simulink model "hw1_sub"  (R2019a)
settings: Solver=VariableStepAuto  StartTime=0.0  StopTime=70  RelTol=1e-12
model workspace (MAT data in the model file):
  d_tar = 20
values from neighbouring files (symbols this model uses):
  d_0 = 8    [acc1.m]
  t_H_tar = 1    [acc1.m]
  v_H0 = 28    [acc1.m]
  v_L0 = 36    [acc1.m]
  v_tar = 36    [acc1.m]
  x_H0 = 0    [acc1.m]
  x_L0 = 50    [acc1.m]
undefined symbols (not defined in the file or in its folder): sigbuilder_block
libraries: cstblocks x3
settings Model: Creator=jake  LastModifiedBy=Lorenzo
settings DebuggingCC: SFMachineParentedDataDiag=error

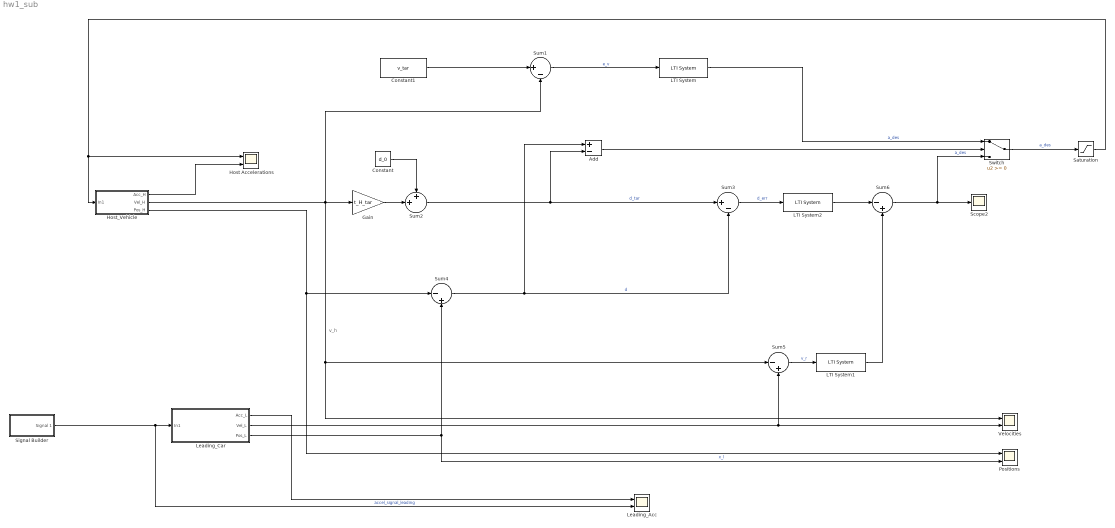
== system hw1_sub ==
  note: v_h
  Add : Sum  Inputs=+-
  Constant : Constant  Value=d_0
  Constant1 : Constant  Value=v_tar
  Gain : Gain  Gain=t_H_tar
  Host Accelerations : Scope  NumInputPorts=2
  Host_Vehicle : Subsystem
  LTI System : cstblocks/LTI System  sys=K_v  IC=[]
  LTI System1 : cstblocks/LTI System  sys=K_v_r  IC=[]
  LTI System2 : cstblocks/LTI System  sys=K_d_err  IC=[]
  Leading_Acc : Scope  NumInputPorts=2
  Leading_Car : Subsystem
  Positions : Scope  NumInputPorts=2
  Saturation : Saturate  UpperLimit=5  LowerLimit=-3
  Scope2 : Scope
  Signal Builder : Subsystem  Tag=STV Subsys  LoadFcn=sigbuilder_block('load');  StartFcn=sigbuilder_block('start');  StopFcn=sigbuilder_block('stop');  ClipboardFcn=sigbuilder_block('clipboard');  mask(Sigbuilder block){tuvar=[0:10]}
      mask help: Simulink:masks:SigbuilderBlock_MD
      mask init:
      | if ~strcmp(get_param(bdroot(gcbh),'SimulationStatus'),'stopped') tuvar = sigbuilder_block('maskInit'); end
      settings: CopyFcn=sigbuilder_block('copy');  DeleteFcn=sigbuilder_block('delete');  ModelCloseFcn=sigbuilder_block('modelClose');  PreSaveFcn=sigbuilder_block('preSave');  PauseFcn=sigbuilder_block('pause');  ContinueFcn=sigbuilder_block('continue');  NameChangeFcn=sigbuilder_block('namechange');  OpenFcn=sigbuilder_block('open',[303 126.6 843.6 459.6 ]);  CloseFcn=sigbuilder_block('close');
      mask Display: plot(0, 0, 100, 100,[2, 2, 32, 32, 2], [68, 8, 8, 68, 68],[32, 2], [38, 38], [32, 19, 2],[53, 60, 44], [32, 17, 17, 2],[16, 16, 31, 31]);txt = getActiveGroup(gcbh);text(2, 100, txt,'verticalAlignment', 'top');
  Sum1 : Sum  Inputs=|+-
  Sum2 : Sum  Inputs=++|
  Sum3 : Sum  Inputs=|+-
  Sum4 : Sum  Inputs=|-+
  Sum5 : Sum  Inputs=|-+
  Sum6 : Sum  Inputs=|-+
  Switch : Switch
  Velocities : Scope  NumInputPorts=2
  wires:
  Leading_Car/3(Pos_L) -> Positions/2, Sum4/2  "x_l"
  Sum1/1 -> LTI System/1  "e_v"
  Gain/1 -> Sum2/2
  Constant/1 -> Sum2/1
  Sum2/1 -> Add/2, Sum3/1  "d_tar"
  Sum4/1 -> Add/1, Sum3/2  "d"
  Sum5/1 -> LTI System1/1  "v_r"
  Sum3/1 -> LTI System2/1  "d_err"
  LTI System1/1 -> Sum6/2
  LTI System2/1 -> Sum6/1
  Sum6/1 -> Switch/3, Scope2/1  "a_des"
  LTI System/1 -> Switch/1  "a_des"
  Constant1/1 -> Sum1/1
  Switch/1 -> Saturation/1  "a_des"
  Signal Builder/1(Signal 1) -> Leading_Acc/2, Leading_Car/1(In1)  "accel_signal_leading"
  Add/1 -> Switch/2
  Leading_Car/2(Vel_L) -> Sum5/2, Velocities/2
  Leading_Car/1(Acc_L) -> Leading_Acc/1
  Host_Vehicle/2(Vel_H) -> Sum5/1, Velocities/1, Sum1/2, Gain/1
  Host_Vehicle/3(Pos_H) -> Positions/1, Sum4/1
  Saturation/1 -> Host Accelerations/1, Host_Vehicle/1(In1)
  Host_Vehicle/1(Acc_H) -> Host Accelerations/2

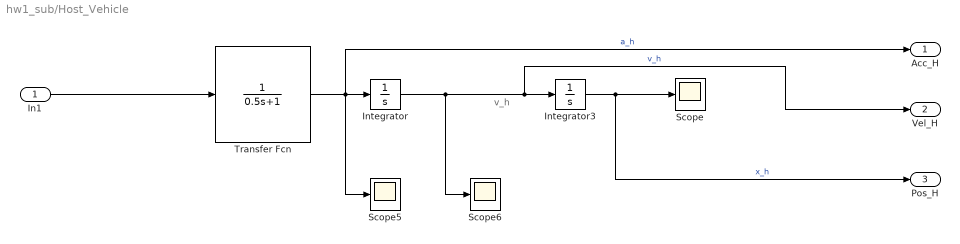
== system hw1_sub/Host_Vehicle ==
  note: v_h
  In1 : Inport
  Integrator : Integrator  InitialCondition=v_H0
  Integrator3 : Integrator  InitialCondition=x_H0
  Scope : Scope
  Scope5 : Scope
  Scope6 : Scope
  Transfer Fcn : TransferFcn  Denominator=[0.5 1]
  Acc_H : Outport
  Vel_H : Outport  Port=2
  Pos_H : Outport  Port=3
  wires:
  Integrator3/1 -> Pos_H/1, Scope/1  "x_h"
  Integrator/1 -> Scope6/1, Vel_H/1, Integrator3/1  "v_h"
  Transfer Fcn/1 -> Acc_H/1, Scope5/1, Integrator/1  "a_h"
  In1/1 -> Transfer Fcn/1

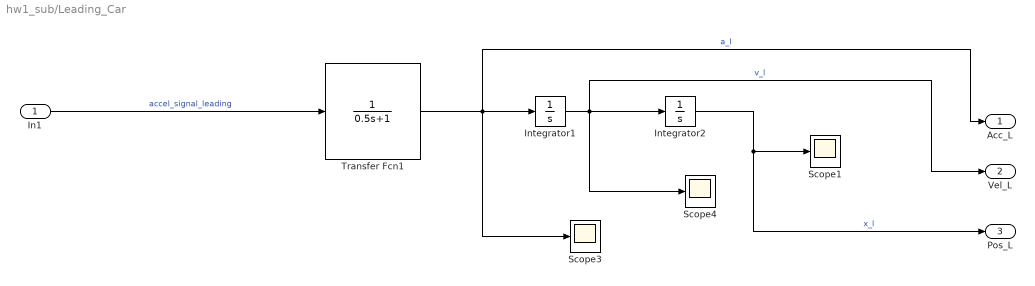
== system hw1_sub/Leading_Car ==
  In1 : Inport
  Integrator1 : Integrator  InitialCondition=v_L0
  Integrator2 : Integrator  InitialCondition=x_L0
  Scope1 : Scope
  Scope3 : Scope
  Scope4 : Scope
  Transfer Fcn1 : TransferFcn  Denominator=[0.5 1]
  Acc_L : Outport
  Vel_L : Outport  Port=2
  Pos_L : Outport  Port=3
  wires:
  Integrator1/1 -> Scope4/1, Vel_L/1, Integrator2/1  "v_l"
  Integrator2/1 -> Pos_L/1, Scope1/1  "x_l"
  Transfer Fcn1/1 -> Scope3/1, Acc_L/1, Integrator1/1  "a_l"
  In1/1 -> Transfer Fcn1/1  "accel_signal_leading"

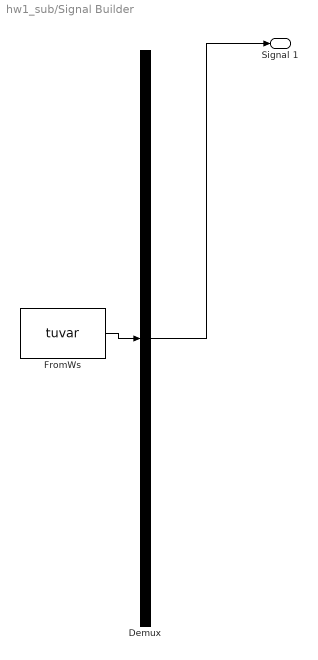
== system hw1_sub/Signal Builder ==
  Demux : Demux  Tag=STV Demux  Outputs=1
      settings: DisplayOption=none
  FromWs : FromWorkspace  Tag=STV FromWs  VariableName=tuvar
      SigBuilderData=|
      | common.afterFinalStr = 'Extrapolate'
      | common.sampleTime = 0
      | dataSet.timeRange = [0 46]
      | dataSet.name = 'Group 1'
      | sbobj.Groups.Name = 'Group 1'
      | sbobj.Groups.Signals.Name = 'Signal 1'
      | sbobj.Groups.Signals.XData = [0 10 10.5 13.5 14 40 40.5 43.5 44 46]
      | sbobj.Groups.Signals.YData = [0 0 -2 -2 0 0 2 2 0 0]
      | sbobj.Groups.TimeRange = [0 46]
  Signal 1 : Outport  Tag=STV Outport
  wires:
  Demux/1 -> Signal 1/1
  FromWs/1 -> Demux/1
